simulink model "gm_spectrum_analyser"  (R2020a)
settings: Solver=VariableStepAuto  StartTime=0.0  StopTime=100000/256e6  RelTol=1e-3
InitFcn:
  | fs = 256e6;
undefined symbols (not defined in the file or in its folder): designMultirateFIR
libraries: hdlsllib x81, simulink x50, dspmlti4 x6, dsphdlxfrm x5, hdlmdlgenlib x4, dspswit3 x4, dspsigops x2, dspsigattribs x2
(part 5 of 5)

== system gm_spectrum_analyser/Spectrum Analyser/Spectrum Analyser/Spectrum Analyser Core/SSR Subset Converter/SSR Serializer Real/SSR4 to SSR8 ==
  Data In : Inport  OutDataTypeStr=uint16  PortDimensions=[8]  SampleTime=3.90625e-09
  Index : Inport  Port=2  OutDataTypeStr=fixdt(0, 1, 0)  PortDimensions=1  SampleTime=3.90625e-09
  Valid In : Inport  Port=3  OutDataTypeStr=boolean  PortDimensions=1  SampleTime=3.90625e-09
  AND : Logic  AllPortsSameDT=off  OutDataTypeStr=boolean  SampleTime=3.90625e-09
  AND1 : Logic  AllPortsSameDT=off  OutDataTypeStr=boolean  SampleTime=3.90625e-09
  Compare To Constant12 : simulink/Logic and Bit Operations/Compare To Constant  relop===  const="fi(0,0,1,0,\"hex\",\"0\")"  OutDataTypeStr=boolean
  Compare To Constant13 : simulink/Logic and Bit Operations/Compare To Constant  relop===  const="fi(0,0,1,0,\"hex\",\"1\")"  OutDataTypeStr=boolean
  Delay : Delay  DelayLength=double(1)  InitialCondition=0  SampleTime=3.90625e-09
  Delay_Switch : Switch  Criteria=u2 ~= 0  Threshold=double(0)  OutDataTypeStr=uint16  SampleTime=3.90625e-09
  Delay_Switch1 : Switch  Criteria=u2 ~= 0  Threshold=double(0)  OutDataTypeStr=uint16  SampleTime=3.90625e-09
  Selector13 : Selector  IndexMode=Zero-based  SampleTime=3.90625e-09  IndexOptions=Index vector (dialog)  Indices=double([0 1 2 3])  OutputSizes=double(1)
  Selector14 : Selector  IndexMode=Zero-based  SampleTime=3.90625e-09  IndexOptions=Index vector (dialog)  Indices=double([0 1 2 3])  OutputSizes=double(1)
  Unit Delay Enabled Synchronous1_lowered : Delay  DelayLength=double(1)  InitialCondition=0  SampleTime=3.90625e-09
  Unit Delay Enabled Synchronous_lowered : Delay  DelayLength=double(1)  InitialCondition=0  SampleTime=3.90625e-09
  concatenate : Concatenate  NumInputs=8
  t : Demux
  t1 : Demux
  Data Out : Outport
  Valid Out : Outport  Port=2
  wires:
  AND/1 -> Delay_Switch/2
  AND1/1 -> Delay/1, Delay_Switch1/2
  Compare To Constant12/1 -> AND/2
  Compare To Constant13/1 -> AND1/2
  Delay/1 -> Valid Out/1
  Selector13/1 -> Delay_Switch/1
  Selector14/1 -> Delay_Switch1/1
  Unit Delay Enabled Synchronous_lowered/1 -> t/1, Delay_Switch/3
  Unit Delay Enabled Synchronous1_lowered/1 -> t1/1, Delay_Switch1/3
  concatenate/1 -> Data Out/1
  t/1 -> concatenate/1
  t/2 -> concatenate/2
  t/3 -> concatenate/3
  t/4 -> concatenate/4
  t1/1 -> concatenate/5
  t1/2 -> concatenate/6
  t1/3 -> concatenate/7
  t1/4 -> concatenate/8
  Data In/1 -> Selector14/1, Selector13/1
  Index/1 -> Compare To Constant13/1, Compare To Constant12/1
  Valid In/1 -> AND1/1, AND/1
  Delay_Switch/1 -> Unit Delay Enabled Synchronous_lowered/1
  Delay_Switch1/1 -> Unit Delay Enabled Synchronous1_lowered/1

== system gm_spectrum_analyser/Spectrum Analyser/Spectrum Analyser/Spectrum Analyser Core/SSR Subset Converter/SSR Serializer Real/Vector to SSR ==
  Vector : Inport  OutDataTypeStr=uint16  PortDimensions=[8]  SampleTime=3.90625e-09
  Bit Concat : hdlsllib/Logic and Bit Operations/Bit Concat  numInputs=8
  Selector0 : Selector  SampleTime=3.90625e-09  IndexOptions=Index vector (dialog)  Indices=double(8)  OutputSizes=double(1)
  Selector1 : Selector  SampleTime=3.90625e-09  IndexOptions=Index vector (dialog)  Indices=double(7)  OutputSizes=double(1)
  Selector2 : Selector  SampleTime=3.90625e-09  IndexOptions=Index vector (dialog)  Indices=double(6)  OutputSizes=double(1)
  Selector3 : Selector  SampleTime=3.90625e-09  IndexOptions=Index vector (dialog)  Indices=double(5)  OutputSizes=double(1)
  Selector4 : Selector  SampleTime=3.90625e-09  IndexOptions=Index vector (dialog)  Indices=double(4)  OutputSizes=double(1)
  Selector5 : Selector  SampleTime=3.90625e-09  IndexOptions=Index vector (dialog)  Indices=double(3)  OutputSizes=double(1)
  Selector6 : Selector  SampleTime=3.90625e-09  IndexOptions=Index vector (dialog)  Indices=double(2)  OutputSizes=double(1)
  Selector7 : Selector  SampleTime=3.90625e-09  IndexOptions=Index vector (dialog)  Indices=double(1)  OutputSizes=double(1)
  SSR : Outport
  wires:
  Bit Concat/1 -> SSR/1
  Selector0/1 -> Bit Concat/1
  Selector1/1 -> Bit Concat/2
  Selector2/1 -> Bit Concat/3
  Selector3/1 -> Bit Concat/4
  Selector4/1 -> Bit Concat/5
  Selector5/1 -> Bit Concat/6
  Selector6/1 -> Bit Concat/7
  Selector7/1 -> Bit Concat/8
  Vector/1 -> Selector7/1, Selector6/1, Selector5/1, Selector4/1, Selector3/1, Selector2/1, Selector1/1, Selector0/1

== system gm_spectrum_analyser/Stimulus and Channel/Channel/RF-ADC/NCO and Mixer/RF-ADC Coarse Mixer/Negate ==
  Data In : Inport
  Complex to Real-Imag2 : ComplexToRealImag
  Real-Imag to Complex1 : RealImagToComplex
  Unary Minus : UnaryMinus
  Data Out : Outport  VectorParamsAs1DForOutWhenUnconnected=off
  wires:
  Complex to Real-Imag2/2 -> Unary Minus/1
  Unary Minus/1 -> Real-Imag to Complex1/2
  Data In/1 -> Complex to Real-Imag2/1
  Real-Imag to Complex1/1 -> Data Out/1
  Complex to Real-Imag2/1 -> Real-Imag to Complex1/1

== system gm_spectrum_analyser/Stimulus and Channel/Channel/RF-ADC/NCO and Mixer/RF-ADC Coarse Mixer/fs_2 ==
  Data In : Inport
  Counter : dspswit3/Counter  Direction=Up  CountEvent=Free running  CounterSize=User defined  MaxCount=1  InitialCount=0  Output=Count  HitValue=32  ResetInput=off  SamplesPerFrame=ssr  Ts=1/(fs)  CntDtype=uint8  HitDtype=Logical
  Multiport Switch2 : MultiPortSwitch  DataPortOrder=Zero-based contiguous  Inputs=2  zeroidx=on
  Real-Imag to Complex : RealImagToComplex
  Real-Imag to Complex1 : RealImagToComplex
  Unary Minus1 : UnaryMinus
  Data Out : Outport  VectorParamsAs1DForOutWhenUnconnected=off
  wires:
  Data In/1 -> Real-Imag to Complex1/1, Real-Imag to Complex1/2, Unary Minus1/1
  Real-Imag to Complex1/1 -> Multiport Switch2/2
  Real-Imag to Complex/1 -> Multiport Switch2/3
  Multiport Switch2/1 -> Data Out/1
  Counter/1 -> Multiport Switch2/1
  Unary Minus1/1 -> Real-Imag to Complex/2, Real-Imag to Complex/1

== system gm_spectrum_analyser/Stimulus and Channel/Channel/RF-ADC/NCO and Mixer/RF-ADC Coarse Mixer/fs_4 ==
  note: Real:	1, 0, -1, 0
      | Imag:	0, 1, 0, -1
  Data In : Inport
  Counter : dspswit3/Counter  Direction=Up  CountEvent=Free running  CounterSize=User defined  MaxCount=3  InitialCount=0  Output=Count  HitValue=32  ResetInput=off  SamplesPerFrame=ssr  Ts=1/(fs)  CntDtype=uint8  HitDtype=Logical
  Multiport Switch2 : MultiPortSwitch  DataPortOrder=Zero-based contiguous  Inputs=4  zeroidx=on
  Real-Imag to Complex{1..4} (4 alike) : RealImagToComplex
  Unary Minus : UnaryMinus
  Unary Minus1 : UnaryMinus
  Unary Minus2 : UnaryMinus
  Data Out : Outport  VectorParamsAs1DForOutWhenUnconnected=off
  wires:
  Unary Minus/1 -> Real-Imag to Complex3/1
  Unary Minus2/1 -> Real-Imag to Complex2/2
  Real-Imag to Complex4/1 -> Multiport Switch2/2
  Unary Minus1/1 -> Real-Imag to Complex1/2, Real-Imag to Complex1/1
  Real-Imag to Complex1/1 -> Multiport Switch2/4
  Counter/1 -> Multiport Switch2/1
  Real-Imag to Complex2/1 -> Multiport Switch2/3
  Data In/1 -> Real-Imag to Complex4/1, Unary Minus2/1, Unary Minus1/1, Unary Minus/1, Real-Imag to Complex3/2, Real-Imag to Complex2/1, Real-Imag to Complex4/2
  Real-Imag to Complex3/1 -> Multiport Switch2/5
  Multiport Switch2/1 -> Data Out/1

== system gm_spectrum_analyser/Stimulus and Channel/Channel/RF-DAC/NCO and Mixer/RF-DAC Coarse Mixer/Negate ==
  Data In : Inport
  Complex to Real-Imag2 : ComplexToRealImag
  Real-Imag to Complex1 : RealImagToComplex
  Unary Minus : UnaryMinus
  Data Out : Outport  VectorParamsAs1DForOutWhenUnconnected=off
  wires:
  Complex to Real-Imag2/1 -> Real-Imag to Complex1/1
  Real-Imag to Complex1/1 -> Data Out/1
  Data In/1 -> Complex to Real-Imag2/1
  Unary Minus/1 -> Real-Imag to Complex1/2
  Complex to Real-Imag2/2 -> Unary Minus/1

== system gm_spectrum_analyser/Stimulus and Channel/Channel/RF-DAC/NCO and Mixer/RF-DAC Coarse Mixer/fs_2 ==
  Data In : Inport
  Counter : dspswit3/Counter  Direction=Up  CountEvent=Free running  CounterSize=User defined  MaxCount=1  InitialCount=0  Output=Count  HitValue=32  ResetInput=off  SamplesPerFrame=ssr  Ts=1/(fs)  CntDtype=uint8  HitDtype=Logical
  Multiport Switch2 : MultiPortSwitch  DataPortOrder=Zero-based contiguous  Inputs=2  zeroidx=on
  Unary Minus : UnaryMinus
  Data Out : Outport  VectorParamsAs1DForOutWhenUnconnected=off
  wires:
  Multiport Switch2/1 -> Data Out/1
  Counter/1 -> Multiport Switch2/1
  Unary Minus/1 -> Multiport Switch2/3
  Data In/1 -> Multiport Switch2/2, Unary Minus/1

== system gm_spectrum_analyser/Stimulus and Channel/Channel/RF-DAC/NCO and Mixer/RF-DAC Coarse Mixer/fs_4 ==
  note: Real:	1, 0, -1, 0
      | Imag:	0, 1, 0, -1
  Data In : Inport
  Complex to Real-Imag : ComplexToRealImag
  Complex to Real-Imag1 : ComplexToRealImag
  Counter : dspswit3/Counter  Direction=Up  CountEvent=Free running  CounterSize=User defined  MaxCount=3  InitialCount=0  Output=Count  HitValue=32  ResetInput=off  SamplesPerFrame=ssr  Ts=1/(fs)  CntDtype=uint8  HitDtype=Logical
  Multiport Switch2 : MultiPortSwitch  DataPortOrder=Zero-based contiguous  Inputs=4  zeroidx=on
  Real-Imag to Complex2 : RealImagToComplex
  Real-Imag to Complex3 : RealImagToComplex
  Unary Minus : UnaryMinus
  Unary Minus1 : UnaryMinus
  Unary Minus2 : UnaryMinus
  Data Out : Outport  VectorParamsAs1DForOutWhenUnconnected=off
  wires:
  Unary Minus2/1 -> Real-Imag to Complex2/1
  Complex to Real-Imag/2 -> Unary Minus2/1
  Unary Minus/1 -> Real-Imag to Complex3/2
  Complex to Real-Imag1/1 -> Unary Minus/1
  Complex to Real-Imag1/2 -> Real-Imag to Complex3/1
  Multiport Switch2/1 -> Data Out/1
  Real-Imag to Complex3/1 -> Multiport Switch2/5
  Data In/1 -> Multiport Switch2/2, Complex to Real-Imag/1, Complex to Real-Imag1/1, Unary Minus1/1
  Unary Minus1/1 -> Multiport Switch2/4
  Complex to Real-Imag/1 -> Real-Imag to Complex2/2
  Real-Imag to Complex2/1 -> Multiport Switch2/3
  Counter/1 -> Multiport Switch2/1

== matlab function gm_spectrum_analyser/DDR Memory/AXI Read Interface Response Model/DDR/Enabled Subsystem/MATLAB Function ==
  data: rd_avalid input; start_counter output; rst input
function start_counter  = fcn(rd_avalid, rst)

persistent start;
if(isempty(start))
    start = false;
end

if (rd_avalid == true)
    start = true;
else
    
    if (rst == true)
        start = false;
    else
        start = start;
    end
end
start_counter = start;

== matlab function gm_spectrum_analyser/Spectrum Analyser/Spectrum Analyser/Direct Memory Access/Direct Memory Access/DDR Communication/Write Controller/slib_spectrum_analyser_c2_Write_Controller ==
  data: valid input; count input; push output boolean; pop output; length input; enable input; start input boolean; wr_complete input; wr_ready input; wr_len output; buffer output; state output; empty input; debug_count output
function [push, pop, wr_len, buffer, state, debug_count] = ddr_write_control(valid, count, length, enable, start, wr_complete, wr_ready, empty)

% Create persistent variables (registers)
persistent burst_count;
persistent time_count;
persistent current_state;
persistent buffer_pointer;

if(isempty(burst_count))
    burst_count = fi(0, 0, 16, 0);
end

if(isempty(time_count))
    time_count = fi(0, 0, 32, 0);
end

if(isempty(current_state))
    current_state = fi(0, 0, 4, 0);
end

if(isempty(buffer_pointer))
    buffer_pointer = fi(0, 0, 2, 0);
end

% FSM States
IDLE  = fi(0, 0, 4, 0);
START = fi(1, 0, 4, 0);
COUNT = fi(2, 0, 4, 0);
WAIT  = fi(4, 0, 4, 0);

switch current_state
    case IDLE
        push = false;
        pop = wr_ready;
        wr_len = length;
        buffer = buffer_pointer;
        state = current_state;
        debug_count = burst_count;
        
        burst_count = fi(0, 0, 16, 0);
        
        if enable && time_count >= count
            current_state = START;
            time_count = fi(0, 0, 32, 0);
        else
            current_state = IDLE;
            if time_count < count
                time_count = fi(time_count + 1, 0, 32, 0);
            end
        end
        
    case START
        pop = false;
        wr_len = length;
        buffer = buffer_pointer;
        state = current_state;
        debug_count = burst_count;
        
        if ~enable
            push = false;
            burst_count = fi(0, 0, 16, 0);
            current_state = IDLE;
        else
            if start && valid
                push = true;
                burst_count = fi(burst_count + 1, 0, 16, 0);
                current_state = COUNT;
            else
                push = false;
                burst_count = fi(0, 0, 16, 0);
                current_state = START;
            end
        end            
        
    case COUNT
        pop = false;
        wr_len = length;
        buffer = buffer_pointer;
        state = current_state;
        debug_count = burst_count;
        
        if valid
            push = true;
            burst_count = fi(burst_count + 1, 0, 16, 0);
        else
            push = false;
        end
        
        if burst_count >= length
            current_state = WAIT;
            if buffer_pointer > fi(1, 0, 2, 0)
                buffer_pointer = fi(0, 0, 2, 0);
            else
            	buffer_pointer = fi(buffer_pointer+1, 0, 2, 0);
            end
        else
            current_state = COUNT;
        end
        
    case WAIT
        push = false;
        pop = wr_ready;
        wr_len = length;
        buffer = buffer_pointer;
        state = current_state;
        debug_count = burst_count;
        
        burst_count = fi(0, 0, 16, 0);
        
        if empty && wr_complete
            current_state = IDLE;
        else
            current_state = WAIT;
        end
        
    otherwise
        push = false;
        pop = wr_ready;
        wr_len = length;
        buffer = buffer_pointer;
        state = current_state;
        debug_count = burst_count;
        
        burst_count = fi(0, 0, 16, 0);
        
        current_state = IDLE;
        
end

== matlab function gm_spectrum_analyser/Spectrum Analyser/Spectrum Analyser/Spectrum Analyser Core/Preprocessing Window/Direct Memory Access/DDR Read Controller/slib_spectrum_analyser_c5_DDR_Read_Controller ==
  data: valid_out output boolean; count_out output; ready_out output boolean; length_in input; address input; start input boolean; rd_aready input; rd_dvalid input; rd_addr output uint32; rd_len output; rd_avalid output
function [valid_out,count_out,ready_out,rd_addr,rd_len,rd_avalid] = ddr_read_control(length_in, address, start, rd_aready, rd_dvalid)

% Create persistent variables (registers)
persistent burst_stop
if(isempty(burst_stop))
    burst_stop = uint16(0);
end
persistent burst_count;
if(isempty(burst_count))
    burst_count = uint16(0);
end
persistent rstate;
if isempty(rstate)
    rstate = fi(0, 0, 4, 0);
end


% State Memory Encoding
IDLE             = fi(1, 0, 4, 0);
READ_BURST_START = fi(2, 0, 4, 0);
DATA_COUNT       = fi(4, 0, 4, 0);

% Read control state machine
switch (rstate)
    case IDLE
        % output to AXI4 Master
        rd_addr = address;
        rd_len = uint16(0);
        rd_avalid = false;
        
        % output to DUT
        valid_out = false;
        ready_out = true;
        count_out = uint16(0);
        
        % State vars
        burst_count = uint16(0);
        burst_stop = uint16(length_in);
        
        if rd_aready && start
            rstate(:) = READ_BURST_START;
        end
        
    case READ_BURST_START
        % output to AXI4 Master
        rd_addr = address;
        rd_len = uint16(burst_stop);
        rd_avalid = true;
        
        % output to DUT
        valid_out = false;
        count_out = uint16(0);
        ready_out = false;
        
        rstate(:) = DATA_COUNT;
        
    case DATA_COUNT
        % output to AXI4 Master
        rd_addr = address;
        rd_len = uint16(burst_stop);
        rd_avalid = false;
        
        % output to DUT
        valid_out = rd_dvalid;
        count_out = uint16(burst_count);
        ready_out = false;
        
        % State vars
        if ( rd_dvalid )
            burst_count = uint16(burst_count + 1);
        end
        
        if ( burst_count == burst_stop )
            rstate(:) = IDLE;
        else
            rstate(:) = DATA_COUNT;
        end
        
    otherwise
        % output to AXI4 Master
        rd_addr = uint32(0);
        rd_len = uint16(0);
        rd_avalid = false;
        
        % output to DUT
        valid_out = false;
        count_out = uint16(0);
        ready_out = false;
        
        rstate(:) = IDLE;
end

end
